simulink model "example4"  (Simulink 7.1)
settings: Solver=ode45  StartTime=0.0  StopTime=Tstop  MaxStep=intg_maxstep  RelTol=1e-6
model workspace: external: M-Code (data not in the file)
undefined symbols (not defined in the file or in its folder): FDfb, singlebody, x_init
libraries: simulink x1
settings Model: Creator=roy  LastModifiedBy=roy
settings DataIOCC: LimitDataPoints=off

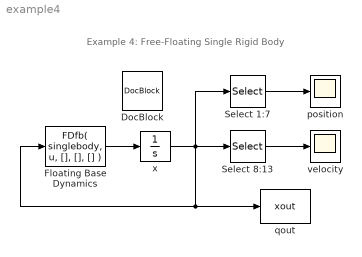
== system example4 ==
  note: Example 4: Free-Floating Single Rigid Body
  DocBlock : simulink/Model-Wide Utilities/DocBlock  SystemSampleTime=-1  DocumentType=Text
      content=|
      | This example shows how to use the function FDfb to simulate a spatial
      | mechanism with a floating base.  The model in this example consists of
      | just a single rigid body.
      |
      | For a spatial rigid-body system, a floating base is modelled as a chain of
      | three prismatic and three revolute joints, all connected together by
      | massless bodies.  This works fine, so long as the floating base does not
      | enter or get very close to the kinematic singularity at q(5) == +/-pi/2.
      | If this happens, or if there is a risk of it happening, then the remedy is
      | to use FDfb instead of FDab.  FDfb works by using a quaternion to
      | represent the orientation of the floating base instead of three joint
      | angles.  To accomplish this, the first six joint position and velocity
      | variables are replaced by a single 13-element state vector, x, which
      | contains a quaternion, a 3D position vector and a spatial velocity, in
      | that order, which describe the orientation, position and velocity of the
      | floating base directly.
      |
      | In this Simulink model, the mechanism being simulated is just a single
      | rigid body, which is tumbling in a zero-gravity environment.  There are
      | therefore no joints in the system other than the six implementing the
      | floating base.  If you open the block "Floating Base Dynamics", you will
      | see the function call "FDfb(singlebody,u,[],[],[])".  In comparison, the
      | calling convention for FDfb is "[xd,qdd]=FDfb(model,x,q,qd,tau,f_ext)".
      | Thus, we can see that the external-force argument has been omitted, that
      | q, qd and tau are all set to empty arrays (because there are no joints
      | other than the ones implementing the floating base), that the input to the
      | block (u) contains only the state vector x, and that the output of the
      | block is the derivative of the state vector, xd.  (Simulink ignores the
      | second output, qdd.)  Thus, the rest of the Simulink model needs only to
      | integrate xd to obtain x, and feed it back to the dynamics calculation
      | block.
      |
      | As there are 13 elements in x, it has been split into 7 position elements
      | and 6 velocity elements for display on two separate scopes.  The vector is
      | also saved to a Matlab workspace variable xout for later processing.
      |
      | Now start the simulation, and watch the signals appear on the two scopes.
      | There is not much that can be immediately deduced from these traces,
      | except that the motion appears to be irregular and non-repetitive in
      | nature.  (In fact it is chaotic. See F. Moon, "Applied Dynamics" to find
      | out why.)  The motion is a bit easier to understand using showmotion.
      | However, showmotion requires a matrix of joint position data as input.
      | Therefore, to see the motion using showmotion, you must use the command
      | "showmotion(singlebody,tout,fbanim(xout))", where fbanim is a special
      | function that converts the position data in xout into the joint data that
      | showmotion needs.
      |
      | When you have finished admiring the motion, you might want to convince
      | yourself that it is correct, or at least accurate.  To help you do this, a
      | special script has been prepared, called ex4_anal, that calculates and
      | plots the drift in the following quantities, all of which are
      | theoretically supposed to be conserved: kinetic energy, position and
      | velocity of centre of mass, and spatial momentum.  Look at the source code
      | to see how it is done.
      |
      | There is one more new item in this example.  If you fire up the model
      | explorer (located in the "View" menu), and take a look at the model
      | workspace for this model (expand "example4" in the "Model Hierarchy" pane
      | (on the left-hand side) and select "Model Workspace"), then you will see
      | that there are several variables defined, and that they have been defined
      | by means of the Matlab code visible in the right-hand panel.  (The crucial
      | detail is the "Data Source" option, which must be set to "M-Code".)  The
      | first two lines define the simulation stop time and maximum integration
      | step size.  (You can see where they are used by clicking on "Configuration
      | Parameters" in the "Simulation" menu in Example 4's window.)  The
      | remaining lines are concerned with calculating x_init, the initial value
      | for x, which appears in the "Initial condition" field of the integration
      | block.
      |
      | You can edit the Matlab code directly, simply by clicking on the panel and
      | typing.  For example, try replacing "vmessy" with "vx", "vy" or "vz" on
      | the line that initializes "v_init".  Once you have made your edit, you
      | must first click on the button marked "Apply", and then on the button
      | "Reinitialize from Source", in order for your changes to take effect.
  Floating Base Dynamics : MATLABFcn  MATLABFcn=FDfb( singlebody, u, [], [], [] )  OutputDimensions=[13 1]  OutputSignalType=real  Output1D=off
  Select 1:7 : Selector  InputPortWidth=13  IndexOptions=Index vector (dialog)  Indices=[1 2 3 4 5 6 7]  OutputSizes=1
  Select 8:13 : Selector  InputPortWidth=13  IndexOptions=Index vector (dialog)  Indices=[8 9 10 11 12 13]  OutputSizes=1
  position : Scope
      settings: YMin=-2  YMax=4
  qout : ToWorkspace  VariableName=xout  SampleTime=-1  SaveFormat=Array
  velocity : Scope
      settings: YMin=-2  YMax=4
  x : Integrator  InitialCondition=x_init
  wires:
  Floating Base Dynamics/1 -> x/1
  Select 1:7/1 -> position/1
  Select 8:13/1 -> velocity/1
  x/1 -> Select 8:13/1, Select 1:7/1, qout/1, Floating Base Dynamics/1
